simulink model "ES101A_DiagcMgrProxyX"  (R2013b)
settings: Solver=ode45  StartTime=0.0  StopTime=10.0  RelTol=1e-3
values from neighbouring files (symbols this model uses):
  DFTAGICNTR_CNT_U08 = DataDict.Constant    [ES101A_DiagcMgr_DataDict.m]
  DIAGCMGR_NTCINFOSTSTESTFAILD_CNT_U08 = DataDict.Constant    [ES101A_DiagcMgr_DataDict.m]
  DIAGCMGR_NTCINFOSTSTESTFAILDTHISIGNCYC_CNT_U08 = DataDict.Constant    [ES101A_DiagcMgr_DataDict.m]
  DIAGCMGR_NTCINFOSTSTESTNOTCMPLTHISIGNCYC_CNT_U08 = DataDict.Constant    [ES101A_DiagcMgr_DataDict.m]
  DiagcMgrFltResp = DataDict.Calibration    [ES101A_DiagcMgr_DataDict.m]
  DIAGCSTSDFTHWAG_CNT_U16 = DataDict.Constant    [ES101A_DiagcMgr_DataDict.m]
  DIAGCSTSDFTHWAGSERLCOMEXPRTVAL_CNT_U16 = DataDict.Constant    [ES101A_DiagcMgr_DataDict.m]
  DIAGCSTSDFTVEHSPD_CNT_U16 = DataDict.Constant    [ES101A_DiagcMgr_DataDict.m]
  DIAGCSTSININVAL_CNT_U16 = DataDict.Constant    [ES101A_DiagcMgr_DataDict.m]
  DIAGCSTSIVTR1INACTV_CNT_U16 = DataDict.Constant    [ES101A_DiagcMgr_DataDict.m]
  DIAGCSTSIVTR2INACTV_CNT_U16 = DataDict.Constant    [ES101A_DiagcMgr_DataDict.m]
  DIAGCSTSLIMDTPRFMNC_CNT_U16 = DataDict.Constant    [ES101A_DiagcMgr_DataDict.m]
  DIAGCSTSWHLIMBREJCTNDI_CNT_U16 = DataDict.Constant    [ES101A_DiagcMgr_DataDict.m]
  ELECGLBPRM_IVTRCNT_CNT_U08 = DataDict.ConfigParam    [ES101A_DiagcMgr_DataDict.m]
  MAXRAMPRATE_ULSPERSEC_F32 = DataDict.Constant    [ES101A_DiagcMgr_DataDict.m]
  MINRAMPRATE_ULSPERSEC_F32 = DataDict.Constant    [ES101A_DiagcMgr_DataDict.m]
  SCAMOTTQCMDTOONE_ULS_F32 = DataDict.Constant    [ES101A_DiagcMgr_DataDict.m]
  SCAMOTTQCMDTOZERO_ULS_F32 = DataDict.Constant    [ES101A_DiagcMgr_DataDict.m]
undefined symbols (not defined in the file or in its folder): ActvMotTqCmdSca, ActvRampRate, AgiCntr, DIAGCMGR_APPLIDXX_CNT_U08, DiagcMgrNtcMap, DiagcSts, NtcStInfo, Sts
libraries: simulink x21
(part 3 of 3)

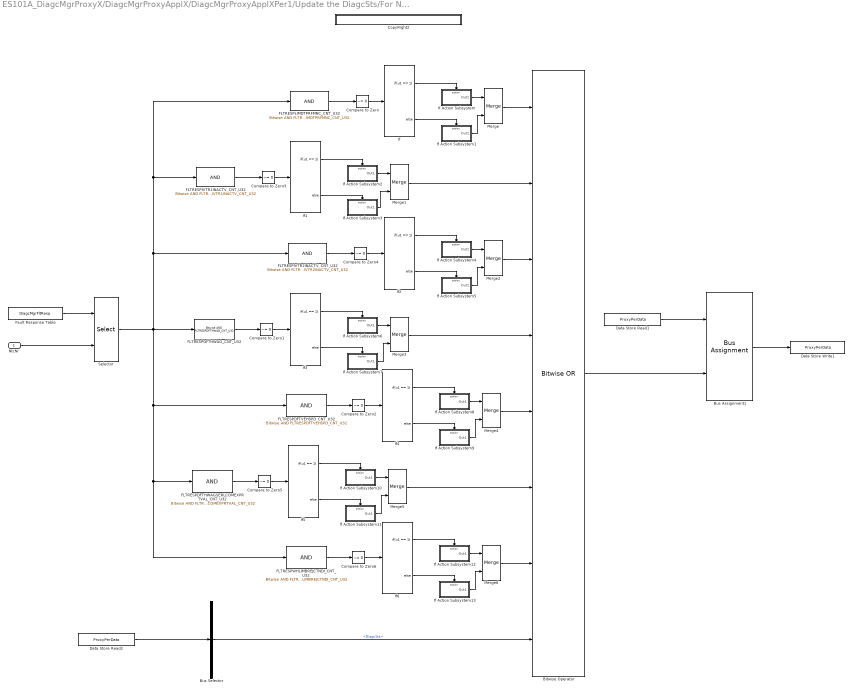
== system ES101A_DiagcMgrProxyX/DiagcMgrProxyApplX/DiagcMgrProxyApplXPer1/Update the DiagcSts/For Number of NTCs/Update DiagcSts and Ramp Response/Update Latest Values/ProcessDiagcSts ==
  NtcNr : Inport
  Bitwise Operator : simulink/Logic and Bit Operations/Bitwise Operator  logicop=OR  UseBitMask=off  NumInputPorts=8  BitMask=bin2dec('11011001')  BitMaskRealWorld=Stored Integer
  Bus Assignment1 : BusAssignment  AssignedSignals=DiagcSts
  Bus Selector : BusSelector  OutputSignals=DiagcSts
  Compare to Zero{,1..6} (7 alike) : simulink/Logic and Bit Operations/Compare To Zero  relop=~=  OutDataTypeStr=boolean
  CopyRight2 : Subsystem  Description=|  mask(Copyright Information){none=on}
      | Copyright info block.                                               
      |                                                                     
      | Place copyright information at the top of every subsystem in design.
      mask prompts: none "No parameters"
      mask help: Place copyright information at the top of every subsystem in design.
      mask Display:
      | NxtrConf = 'Nexteer Confidential';
      | 
      | sys = bdroot; %handle for the current model ("system")
      | first = get_param(sys,'Created');
      | first = first(end-3:end);  %year is last four digits
      | 
      | last = get_param(sys,'LastModifiedDate');
      | if isempty(last)
      |     last = datestr(now,'yyyy');
      | else
      |     last = last(end-3:end);
      | end
      | 
      | if strcmp(first,last)
      |     fprintf('%s -- Copyright %s Nexteer',NxtrConf,first)
      | else
      |     fprintf('%s -- %s%s- %s Nexteer',NxtrConf,char(169),first,last)
      | end
  Data Store Read1 : DataStoreRead  DataStoreName=ProxyPerData
  Data Store Read2 : DataStoreRead  DataStoreName=ProxyPerData
  Data Store Write1 : DataStoreWrite  DataStoreName=ProxyPerData
  FLTRESPDFTHWAGSERLCOMEXPRTVAL_CNT_U32 : simulink/Logic and Bit Operations/Bitwise Operator  logicop=AND  UseBitMask=on  BitMask=FLTRESPDFTHWAGSERLCOMEXPRTVAL_CNT_U32  BitMaskRealWorld=Stored Integer
  FLTRESPDFTHWAG_CNT_U32 : simulink/Logic and Bit Operations/Bitwise Operator  logicop=AND  UseBitMask=on  BitMask=FLTRESPDFTHWAG_CNT_U32  BitMaskRealWorld=Stored Integer
  FLTRESPDFTVEHSPD_CNT_U32 : simulink/Logic and Bit Operations/Bitwise Operator  logicop=AND  UseBitMask=on  BitMask=FLTRESPDFTVEHSPD_CNT_U32  BitMaskRealWorld=Stored Integer
  FLTRESPIVTR1INACTV_CNT_U32 : simulink/Logic and Bit Operations/Bitwise Operator  RequirementInfo={} %GIDa_f3ee0b00_0af4_4caf_9c85_8da4f7631b2d  logicop=AND  UseBitMask=on  BitMask=FLTRESPIVTR1INACTV_CNT_U32  BitMaskRealWorld=Stored Integer
  FLTRESPIVTR2INACTV_CNT_U32 : simulink/Logic and Bit Operations/Bitwise Operator  RequirementInfo={} %GIDa_c098454a_7649_4588_93b4_e3f297a380c8  logicop=AND  UseBitMask=on  BitMask=FLTRESPIVTR2INACTV_CNT_U32  BitMaskRealWorld=Stored Integer
  FLTRESPLIMDTPRFMNC_CNT_U32 : simulink/Logic and Bit Operations/Bitwise Operator  RequirementInfo={} %GIDa_abf10c00_ccc5_4fac_90af_e726bdec96c5  logicop=AND  UseBitMask=on  BitMask=FLTRESPLIMDTPRFMNC_CNT_U32  BitMaskRealWorld=Stored Integer
  FLTRESPWHLIMBREJCTNDI_CNT_U32 : simulink/Logic and Bit Operations/Bitwise Operator  logicop=AND  UseBitMask=on  BitMask=FLTRESPWHLIMBREJCTNDI_CNT_U32  BitMaskRealWorld=Stored Integer
  Fault Response Table : Constant  Value=DiagcMgrFltResp
  If{,1..6} (7 alike) : If  IfExpression=u1 == 1
  If Action Subsystem : Subsystem  TreatAsAtomicUnit=on
  If Action Subsystem1 : Subsystem  TreatAsAtomicUnit=on
  If Action Subsystem10 : Subsystem  TreatAsAtomicUnit=on
  If Action Subsystem11 : Subsystem  TreatAsAtomicUnit=on
  If Action Subsystem12 : Subsystem  TreatAsAtomicUnit=on
  If Action Subsystem13 : Subsystem  TreatAsAtomicUnit=on
  If Action Subsystem2 : Subsystem  TreatAsAtomicUnit=on
  If Action Subsystem3 : Subsystem  TreatAsAtomicUnit=on
  If Action Subsystem4 : Subsystem  TreatAsAtomicUnit=on
  If Action Subsystem5 : Subsystem  TreatAsAtomicUnit=on
  If Action Subsystem6 : Subsystem  TreatAsAtomicUnit=on
  If Action Subsystem7 : Subsystem  TreatAsAtomicUnit=on
  If Action Subsystem8 : Subsystem  TreatAsAtomicUnit=on
  If Action Subsystem9 : Subsystem  TreatAsAtomicUnit=on
  Merge{,1..6} (7 alike) : Merge
  Selector : Selector  IndexMode=Zero-based  InputPortWidth=512  IndexOptions=Index vector (port)  Indices=[1 3]  OutputSizes=1
  wires:
  Bitwise Operator/1 -> Bus Assignment1/2
  Bus Selector/1 -> Bitwise Operator/8  "<DiagcSts>"
  FLTRESPWHLIMBREJCTNDI_CNT_U32/1 -> Compare to Zero6/1
  If6/1 -> If Action Subsystem12/Action
  If6/2 -> If Action Subsystem13/Action
  If Action Subsystem12/1(Out1) -> Merge6/1
  If Action Subsystem13/1(Out1) -> Merge6/2
  Merge6/1 -> Bitwise Operator/7
  Compare to Zero6/1 -> If6/1
  FLTRESPDFTHWAGSERLCOMEXPRTVAL_CNT_U32/1 -> Compare to Zero5/1
  If5/1 -> If Action Subsystem10/Action
  If5/2 -> If Action Subsystem11/Action
  If Action Subsystem10/1(Out1) -> Merge5/1
  If Action Subsystem11/1(Out1) -> Merge5/2
  Merge5/1 -> Bitwise Operator/6
  Compare to Zero5/1 -> If5/1
  FLTRESPDFTVEHSPD_CNT_U32/1 -> Compare to Zero2/1
  If4/1 -> If Action Subsystem8/Action
  If4/2 -> If Action Subsystem9/Action
  If Action Subsystem8/1(Out1) -> Merge4/1
  If Action Subsystem9/1(Out1) -> Merge4/2
  Merge4/1 -> Bitwise Operator/5
  Compare to Zero2/1 -> If4/1
  FLTRESPDFTHWAG_CNT_U32/1 -> Compare to Zero1/1
  If3/1 -> If Action Subsystem6/Action
  If3/2 -> If Action Subsystem7/Action
  If Action Subsystem6/1(Out1) -> Merge3/1
  If Action Subsystem7/1(Out1) -> Merge3/2
  Merge3/1 -> Bitwise Operator/4
  Compare to Zero1/1 -> If3/1
  FLTRESPLIMDTPRFMNC_CNT_U32/1 -> Compare to Zero/1
  NtcNr/1 -> Selector/2
  Fault Response Table/1 -> Selector/1
  Selector/1 -> FLTRESPIVTR2INACTV_CNT_U32/1, FLTRESPIVTR1INACTV_CNT_U32/1, FLTRESPLIMDTPRFMNC_CNT_U32/1, FLTRESPDFTHWAG_CNT_U32/1, FLTRESPDFTVEHSPD_CNT_U32/1, FLTRESPDFTHWAGSERLCOMEXPRTVAL_CNT_U32/1, FLTRESPWHLIMBREJCTNDI_CNT_U32/1
  FLTRESPIVTR1INACTV_CNT_U32/1 -> Compare to Zero3/1
  FLTRESPIVTR2INACTV_CNT_U32/1 -> Compare to Zero4/1
  If/1 -> If Action Subsystem/Action
  If/2 -> If Action Subsystem1/Action
  Compare to Zero/1 -> If/1
  If Action Subsystem/1(Out1) -> Merge/1
  If Action Subsystem1/1(Out1) -> Merge/2
  Merge/1 -> Bitwise Operator/1
  If1/1 -> If Action Subsystem2/Action
  If1/2 -> If Action Subsystem3/Action
  If Action Subsystem2/1(Out1) -> Merge1/1
  If Action Subsystem3/1(Out1) -> Merge1/2
  Compare to Zero3/1 -> If1/1
  Merge1/1 -> Bitwise Operator/2
  If2/1 -> If Action Subsystem4/Action
  If2/2 -> If Action Subsystem5/Action
  If Action Subsystem4/1(Out1) -> Merge2/1
  If Action Subsystem5/1(Out1) -> Merge2/2
  Merge2/1 -> Bitwise Operator/3
  Compare to Zero4/1 -> If2/1
  Data Store Read1/1 -> Bus Assignment1/1
  Bus Assignment1/1 -> Data Store Write1/1
  Data Store Read2/1 -> Bus Selector/1

== system ES101A_DiagcMgrProxyX/DiagcMgrProxyApplX/DiagcMgrProxyApplXPer1/Update the DiagcSts/For Number of NTCs/Update DiagcSts and Ramp Response/Update Latest Values/ProcessRampResponse ==
  NtcNr : Inport
  Arithmetic Right Shift : ArithShift  BitShiftNumber=8  BitShiftDirection=Right
  ControlledShutdown Fault : Subsystem  RequirementInfo={} %GIDa_725417ca_b856_44d5_8006_295b90ff6843  TreatAsAtomicUnit=on
  CopyRight2 : Subsystem  Description=|  mask(Copyright Information){none=on}
      | Copyright info block.                                               
      |                                                                     
      | Place copyright information at the top of every subsystem in design.
      mask prompts: none "No parameters"
      mask help: Place copyright information at the top of every subsystem in design.
      mask Display:
      | NxtrConf = 'Nexteer Confidential';
      | 
      | sys = bdroot; %handle for the current model ("system")
      | first = get_param(sys,'Created');
      | first = first(end-3:end);  %year is last four digits
      | 
      | last = get_param(sys,'LastModifiedDate');
      | if isempty(last)
      |     last = datestr(now,'yyyy');
      | else
      |     last = last(end-3:end);
      | end
      | 
      | if strcmp(first,last)
      |     fprintf('%s -- Copyright %s Nexteer',NxtrConf,first)
      | else
      |     fprintf('%s -- %s%s- %s Nexteer',NxtrConf,char(169),first,last)
      | end
  FLTRESPRAMPBITS_CNT_U32 : simulink/Logic and Bit Operations/Bitwise Operator  logicop=AND  UseBitMask=on  BitMask=FLTRESPRAMPBITS_CNT_U32  BitMaskRealWorld=Stored Integer
  Fault Response Table : Constant  Value=DiagcMgrFltResp
  InformationOnly Fault : Subsystem  RequirementInfo={} %GIDa_ae2e5ce0_c467_4af9_b6e8_59d2bb6bb901  TreatAsAtomicUnit=on
  RapidShutdown Fault : Subsystem  RequirementInfo={} %GIDa_75af6023_41ae_4178_91eb_a83436bbf5a3  TreatAsAtomicUnit=on
  Selector1 : Selector  IndexMode=Zero-based  InputPortWidth=512  IndexOptions=Index vector (port)  Indices=[1 3]  OutputSizes=1
  Switch Case : SwitchCase  CaseConditions={15,14,13}
  TimedShutdown Fault : Subsystem  RequirementInfo={} %GIDa_32e9e7ae_b862_4160_9cdf_f89576b3a813  TreatAsAtomicUnit=on
  wires:
  Switch Case/4 -> TimedShutdown Fault/Action
  Switch Case/3 -> RapidShutdown Fault/Action
  Switch Case/2 -> ControlledShutdown Fault/Action
  Switch Case/1 -> InformationOnly Fault/Action
  Fault Response Table/1 -> Selector1/1
  Selector1/1 -> FLTRESPRAMPBITS_CNT_U32/1
  FLTRESPRAMPBITS_CNT_U32/1 -> Arithmetic Right Shift/1
  Arithmetic Right Shift/1 -> Switch Case/1, TimedShutdown Fault/1(FaultResponseRampBits)
  NtcNr/1 -> Selector1/2

== system ES101A_DiagcMgrProxyX/DiagcMgrProxyApplX/DiagcMgrProxyApplXPer1/Update the DiagcSts/For Number of NTCs/Update DiagcSts and Ramp Response/Update Latest Values/ProcessDiagcSts/CopyRight2 ==

== system ES101A_DiagcMgrProxyX/DiagcMgrProxyApplX/DiagcMgrProxyApplXPer1/Update the DiagcSts/For Number of NTCs/Update DiagcSts and Ramp Response/Update Latest Values/ProcessDiagcSts/If Action Subsystem ==
  Action Port : ActionPort
  Constant1 : Constant  Value=DIAGCSTSLIMDTPRFMNC_CNT_U16
  Out1 : Outport
  wires:
  Constant1/1 -> Out1/1

== system ES101A_DiagcMgrProxyX/DiagcMgrProxyApplX/DiagcMgrProxyApplXPer1/Update the DiagcSts/For Number of NTCs/Update DiagcSts and Ramp Response/Update Latest Values/ProcessDiagcSts/If Action Subsystem1 ==
  Action Port : ActionPort
  Constant1 : Constant  Value=0  OutDataTypeStr=uint16
  Out1 : Outport
  wires:
  Constant1/1 -> Out1/1

== system ES101A_DiagcMgrProxyX/DiagcMgrProxyApplX/DiagcMgrProxyApplXPer1/Update the DiagcSts/For Number of NTCs/Update DiagcSts and Ramp Response/Update Latest Values/ProcessDiagcSts/If Action Subsystem10 ==
  Action Port : ActionPort
  Constant1 : Constant  Value=DIAGCSTSDFTHWAGSERLCOMEXPRTVAL_CNT_U16
  Out1 : Outport
  wires:
  Constant1/1 -> Out1/1

== system ES101A_DiagcMgrProxyX/DiagcMgrProxyApplX/DiagcMgrProxyApplXPer1/Update the DiagcSts/For Number of NTCs/Update DiagcSts and Ramp Response/Update Latest Values/ProcessDiagcSts/If Action Subsystem11 ==
  Action Port : ActionPort
  Constant1 : Constant  Value=0  OutDataTypeStr=uint16
  Out1 : Outport
  wires:
  Constant1/1 -> Out1/1

== system ES101A_DiagcMgrProxyX/DiagcMgrProxyApplX/DiagcMgrProxyApplXPer1/Update the DiagcSts/For Number of NTCs/Update DiagcSts and Ramp Response/Update Latest Values/ProcessDiagcSts/If Action Subsystem12 ==
  Action Port : ActionPort
  Constant1 : Constant  Value=DIAGCSTSWHLIMBREJCTNDI_CNT_U16
  Out1 : Outport
  wires:
  Constant1/1 -> Out1/1

== system ES101A_DiagcMgrProxyX/DiagcMgrProxyApplX/DiagcMgrProxyApplXPer1/Update the DiagcSts/For Number of NTCs/Update DiagcSts and Ramp Response/Update Latest Values/ProcessDiagcSts/If Action Subsystem13 ==
  Action Port : ActionPort
  Constant1 : Constant  Value=0  OutDataTypeStr=uint16
  Out1 : Outport
  wires:
  Constant1/1 -> Out1/1

== system ES101A_DiagcMgrProxyX/DiagcMgrProxyApplX/DiagcMgrProxyApplXPer1/Update the DiagcSts/For Number of NTCs/Update DiagcSts and Ramp Response/Update Latest Values/ProcessDiagcSts/If Action Subsystem2 ==
  Action Port : ActionPort
  Constant1 : Constant  Value=DIAGCSTSIVTR1INACTV_CNT_U16
  Out1 : Outport
  wires:
  Constant1/1 -> Out1/1

== system ES101A_DiagcMgrProxyX/DiagcMgrProxyApplX/DiagcMgrProxyApplXPer1/Update the DiagcSts/For Number of NTCs/Update DiagcSts and Ramp Response/Update Latest Values/ProcessDiagcSts/If Action Subsystem3 ==
  Action Port : ActionPort
  Constant1 : Constant  Value=0  OutDataTypeStr=uint16
  Out1 : Outport
  wires:
  Constant1/1 -> Out1/1

== system ES101A_DiagcMgrProxyX/DiagcMgrProxyApplX/DiagcMgrProxyApplXPer1/Update the DiagcSts/For Number of NTCs/Update DiagcSts and Ramp Response/Update Latest Values/ProcessDiagcSts/If Action Subsystem4 ==
  Action Port : ActionPort
  Constant1 : Constant  Value=DIAGCSTSIVTR2INACTV_CNT_U16
  Out1 : Outport
  wires:
  Constant1/1 -> Out1/1

== system ES101A_DiagcMgrProxyX/DiagcMgrProxyApplX/DiagcMgrProxyApplXPer1/Update the DiagcSts/For Number of NTCs/Update DiagcSts and Ramp Response/Update Latest Values/ProcessDiagcSts/If Action Subsystem5 ==
  Action Port : ActionPort
  Constant1 : Constant  Value=0  OutDataTypeStr=uint16
  Out1 : Outport
  wires:
  Constant1/1 -> Out1/1

== system ES101A_DiagcMgrProxyX/DiagcMgrProxyApplX/DiagcMgrProxyApplXPer1/Update the DiagcSts/For Number of NTCs/Update DiagcSts and Ramp Response/Update Latest Values/ProcessDiagcSts/If Action Subsystem6 ==
  Action Port : ActionPort
  Constant1 : Constant  Value=DIAGCSTSDFTHWAG_CNT_U16
  Out1 : Outport
  wires:
  Constant1/1 -> Out1/1

== system ES101A_DiagcMgrProxyX/DiagcMgrProxyApplX/DiagcMgrProxyApplXPer1/Update the DiagcSts/For Number of NTCs/Update DiagcSts and Ramp Response/Update Latest Values/ProcessDiagcSts/If Action Subsystem7 ==
  Action Port : ActionPort
  Constant1 : Constant  Value=0  OutDataTypeStr=uint16
  Out1 : Outport
  wires:
  Constant1/1 -> Out1/1

== system ES101A_DiagcMgrProxyX/DiagcMgrProxyApplX/DiagcMgrProxyApplXPer1/Update the DiagcSts/For Number of NTCs/Update DiagcSts and Ramp Response/Update Latest Values/ProcessDiagcSts/If Action Subsystem8 ==
  Action Port : ActionPort
  Constant1 : Constant  Value=DIAGCSTSDFTVEHSPD_CNT_U16
  Out1 : Outport
  wires:
  Constant1/1 -> Out1/1

== system ES101A_DiagcMgrProxyX/DiagcMgrProxyApplX/DiagcMgrProxyApplXPer1/Update the DiagcSts/For Number of NTCs/Update DiagcSts and Ramp Response/Update Latest Values/ProcessDiagcSts/If Action Subsystem9 ==
  Action Port : ActionPort
  Constant1 : Constant  Value=0  OutDataTypeStr=uint16
  Out1 : Outport
  wires:
  Constant1/1 -> Out1/1

== system ES101A_DiagcMgrProxyX/DiagcMgrProxyApplX/DiagcMgrProxyApplXPer1/Update the DiagcSts/For Number of NTCs/Update DiagcSts and Ramp Response/Update Latest Values/ProcessRampResponse/ControlledShutdown Fault ==
  Action Port : ActionPort
  Bus Selector : BusSelector  OutputSignals=ActvMotTqCmdSca
  CopyRight2 : Subsystem  Description=|  mask(Copyright Information){none=on}
      | Copyright info block.                                               
      |                                                                     
      | Place copyright information at the top of every subsystem in design.
      mask prompts: none "No parameters"
      mask help: Place copyright information at the top of every subsystem in design.
      mask Display:
      | NxtrConf = 'Nexteer Confidential';
      | 
      | sys = bdroot; %handle for the current model ("system")
      | first = get_param(sys,'Created');
      | first = first(end-3:end);  %year is last four digits
      | 
      | last = get_param(sys,'LastModifiedDate');
      | if isempty(last)
      |     last = datestr(now,'yyyy');
      | else
      |     last = last(end-3:end);
      | end
      | 
      | if strcmp(first,last)
      |     fprintf('%s -- Copyright %s Nexteer',NxtrConf,first)
      | else
      |     fprintf('%s -- %s%s- %s Nexteer',NxtrConf,char(169),first,last)
      | end
  Data Store Read : DataStoreRead  DataStoreName=ProxyPerData
  Do Nothing : Subsystem  TreatAsAtomicUnit=on
  If : If  NumInputs=2  IfExpression=u1 < u2
  Scale Motor Torque Command to Zero1 : Constant  Value=SCAMOTTQCMDTOZERO_ULS_F32  OutDataTypeStr=single
  Update Scale : Subsystem  TreatAsAtomicUnit=on
  wires:
  Scale Motor Torque Command to Zero1/1 -> If/1
  Bus Selector/1 -> If/2  "<ActvMotTqCmdSca>"
  If/2 -> Do Nothing/Action
  If/1 -> Update Scale/Action
  Data Store Read/1 -> Bus Selector/1

== system ES101A_DiagcMgrProxyX/DiagcMgrProxyApplX/DiagcMgrProxyApplXPer1/Update the DiagcSts/For Number of NTCs/Update DiagcSts and Ramp Response/Update Latest Values/ProcessRampResponse/CopyRight2 ==

== system ES101A_DiagcMgrProxyX/DiagcMgrProxyApplX/DiagcMgrProxyApplXPer1/Update the DiagcSts/For Number of NTCs/Update DiagcSts and Ramp Response/Update Latest Values/ProcessRampResponse/InformationOnly Fault ==
  Action Port : ActionPort
  CopyRight2 : Subsystem  Description=|  mask(Copyright Information){none=on}
      | Copyright info block.                                               
      |                                                                     
      | Place copyright information at the top of every subsystem in design.
      mask prompts: none "No parameters"
      mask help: Place copyright information at the top of every subsystem in design.
      mask Display:
      | NxtrConf = 'Nexteer Confidential';
      | 
      | sys = bdroot; %handle for the current model ("system")
      | first = get_param(sys,'Created');
      | first = first(end-3:end);  %year is last four digits
      | 
      | last = get_param(sys,'LastModifiedDate');
      | if isempty(last)
      |     last = datestr(now,'yyyy');
      | else
      |     last = last(end-3:end);
      | end
      | 
      | if strcmp(first,last)
      |     fprintf('%s -- Copyright %s Nexteer',NxtrConf,first)
      | else
      |     fprintf('%s -- %s%s- %s Nexteer',NxtrConf,char(169),first,last)
      | end

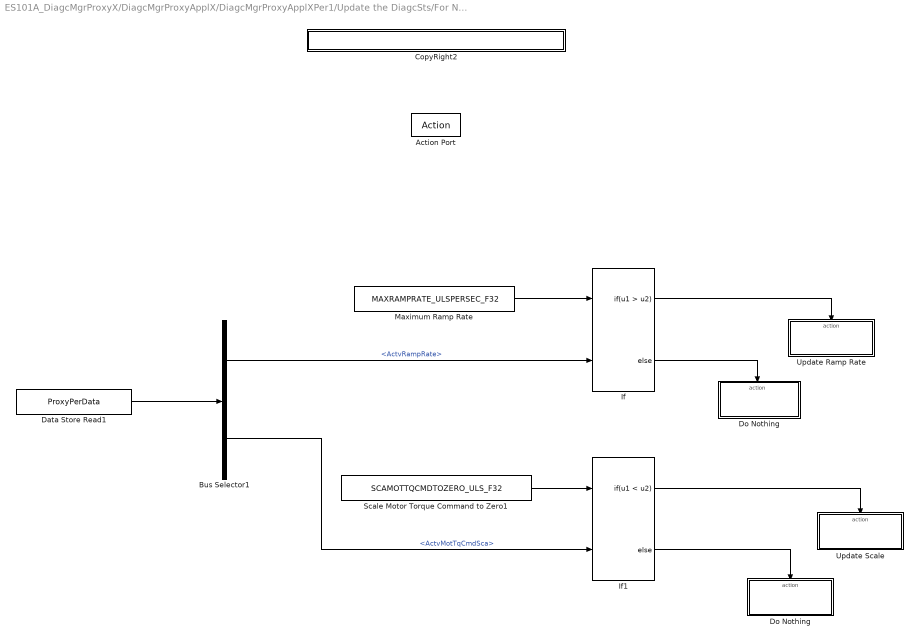
== system ES101A_DiagcMgrProxyX/DiagcMgrProxyApplX/DiagcMgrProxyApplXPer1/Update the DiagcSts/For Number of NTCs/Update DiagcSts and Ramp Response/Update Latest Values/ProcessRampResponse/RapidShutdown Fault ==
  Action Port : ActionPort
  Bus Selector1 : BusSelector  OutputSignals=ActvRampRate,ActvMotTqCmdSca
  CopyRight2 : Subsystem  Description=|  mask(Copyright Information){none=on}
      | Copyright info block.                                               
      |                                                                     
      | Place copyright information at the top of every subsystem in design.
      mask prompts: none "No parameters"
      mask help: Place copyright information at the top of every subsystem in design.
      mask Display:
      | NxtrConf = 'Nexteer Confidential';
      | 
      | sys = bdroot; %handle for the current model ("system")
      | first = get_param(sys,'Created');
      | first = first(end-3:end);  %year is last four digits
      | 
      | last = get_param(sys,'LastModifiedDate');
      | if isempty(last)
      |     last = datestr(now,'yyyy');
      | else
      |     last = last(end-3:end);
      | end
      | 
      | if strcmp(first,last)
      |     fprintf('%s -- Copyright %s Nexteer',NxtrConf,first)
      | else
      |     fprintf('%s -- %s%s- %s Nexteer',NxtrConf,char(169),first,last)
      | end
  Data Store Read1 : DataStoreRead  DataStoreName=ProxyPerData
  Do Nothing : Subsystem  TreatAsAtomicUnit=on
  "Do Nothing " : Subsystem  TreatAsAtomicUnit=on
  If : If  NumInputs=2  IfExpression=u1 > u2
  If1 : If  NumInputs=2  IfExpression=u1 < u2
  Maximum Ramp Rate : Constant  Value=MAXRAMPRATE_ULSPERSEC_F32  OutDataTypeStr=single
  Scale Motor Torque Command to Zero1 : Constant  Value=SCAMOTTQCMDTOZERO_ULS_F32  OutDataTypeStr=single
  Update Ramp Rate : Subsystem  TreatAsAtomicUnit=on
  Update Scale : Subsystem  TreatAsAtomicUnit=on
  wires:
  Maximum Ramp Rate/1 -> If/1
  Bus Selector1/1 -> If/2  "<ActvRampRate>"
  If/2 -> "Do Nothing "/Action
  If/1 -> Update Ramp Rate/Action
  Scale Motor Torque Command to Zero1/1 -> If1/1
  If1/2 -> Do Nothing/Action
  If1/1 -> Update Scale/Action
  Data Store Read1/1 -> Bus Selector1/1
  Bus Selector1/2 -> If1/2  "<ActvMotTqCmdSca>"

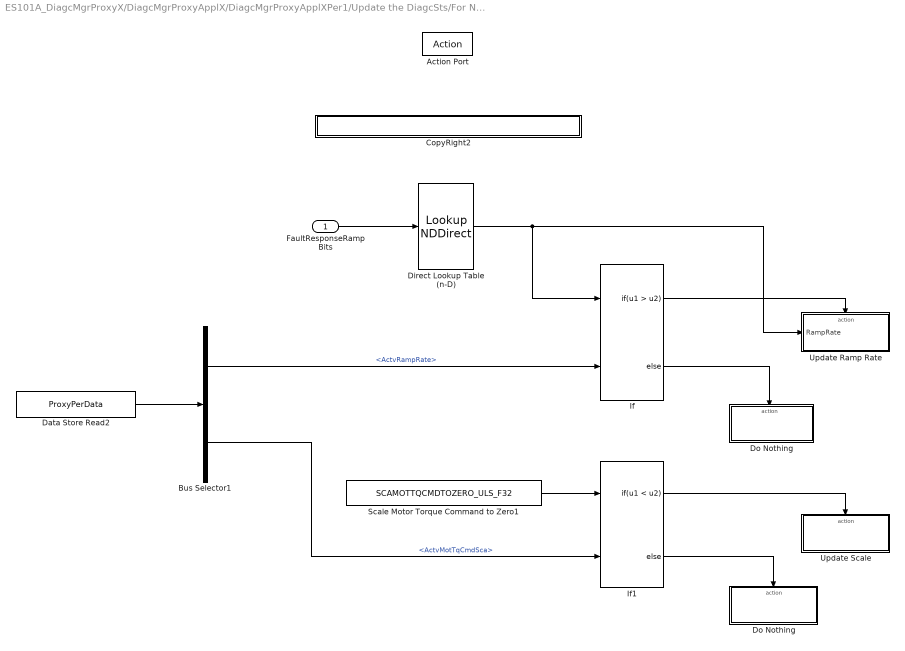
== system ES101A_DiagcMgrProxyX/DiagcMgrProxyApplX/DiagcMgrProxyApplXPer1/Update the DiagcSts/For Number of NTCs/Update DiagcSts and Ramp Response/Update Latest Values/ProcessRampResponse/TimedShutdown Fault ==
  FaultResponseRampBits : Inport
  Action Port : ActionPort
  Bus Selector1 : BusSelector  OutputSignals=ActvRampRate,ActvMotTqCmdSca
  CopyRight2 : Subsystem  Description=|  mask(Copyright Information){none=on}
      | Copyright info block.                                               
      |                                                                     
      | Place copyright information at the top of every subsystem in design.
      mask prompts: none "No parameters"
      mask help: Place copyright information at the top of every subsystem in design.
      mask Display:
      | NxtrConf = 'Nexteer Confidential';
      | 
      | sys = bdroot; %handle for the current model ("system")
      | first = get_param(sys,'Created');
      | first = first(end-3:end);  %year is last four digits
      | 
      | last = get_param(sys,'LastModifiedDate');
      | if isempty(last)
      |     last = datestr(now,'yyyy');
      | else
      |     last = last(end-3:end);
      | end
      | 
      | if strcmp(first,last)
      |     fprintf('%s -- Copyright %s Nexteer',NxtrConf,first)
      | else
      |     fprintf('%s -- %s%s- %s Nexteer',NxtrConf,char(169),first,last)
      | end
  Data Store Read2 : DataStoreRead  DataStoreName=ProxyPerData
  Direct Lookup Table (n-D) : LookupNDDirect  NumberOfTableDimensions=1  Table=[0.1,0.125,0.1428,0.1667,0.2,0.25,0.333,0.5,1,2,3.333,10,500]  TableDataTypeStr=single
  Do Nothing : Subsystem  TreatAsAtomicUnit=on
  "Do Nothing " : Subsystem  TreatAsAtomicUnit=on
  If : If  NumInputs=2  IfExpression=u1 > u2
  If1 : If  NumInputs=2  IfExpression=u1 < u2
  Scale Motor Torque Command to Zero1 : Constant  Value=SCAMOTTQCMDTOZERO_ULS_F32  OutDataTypeStr=single
  Update Ramp Rate : Subsystem  TreatAsAtomicUnit=on
  Update Scale : Subsystem  TreatAsAtomicUnit=on
  wires:
  Direct Lookup Table (n-D)/1 -> If/1, Update Ramp Rate/1(RampRate)
  Scale Motor Torque Command to Zero1/1 -> If1/1
  If1/2 -> Do Nothing/Action
  If1/1 -> Update Scale/Action
  If/2 -> "Do Nothing "/Action
  If/1 -> Update Ramp Rate/Action
  FaultResponseRampBits/1 -> Direct Lookup Table (n-D)/1
  Bus Selector1/1 -> If/2  "<ActvRampRate>"
  Data Store Read2/1 -> Bus Selector1/1
  Bus Selector1/2 -> If1/2  "<ActvMotTqCmdSca>"

== system ES101A_DiagcMgrProxyX/DiagcMgrProxyApplX/DiagcMgrProxyApplXPer1/Update the DiagcSts/For Number of NTCs/Update DiagcSts and Ramp Response/Update Latest Values/ProcessRampResponse/ControlledShutdown Fault/CopyRight2 ==

== system ES101A_DiagcMgrProxyX/DiagcMgrProxyApplX/DiagcMgrProxyApplXPer1/Update the DiagcSts/For Number of NTCs/Update DiagcSts and Ramp Response/Update Latest Values/ProcessRampResponse/ControlledShutdown Fault/Do Nothing ==
  Action Port : ActionPort
  CopyRight2 : Subsystem  Description=|  mask(Copyright Information){none=on}
      | Copyright info block.                                               
      |                                                                     
      | Place copyright information at the top of every subsystem in design.
      mask prompts: none "No parameters"
      mask help: Place copyright information at the top of every subsystem in design.
      mask Display:
      | NxtrConf = 'Nexteer Confidential';
      | 
      | sys = bdroot; %handle for the current model ("system")
      | first = get_param(sys,'Created');
      | first = first(end-3:end);  %year is last four digits
      | 
      | last = get_param(sys,'LastModifiedDate');
      | if isempty(last)
      |     last = datestr(now,'yyyy');
      | else
      |     last = last(end-3:end);
      | end
      | 
      | if strcmp(first,last)
      |     fprintf('%s -- Copyright %s Nexteer',NxtrConf,first)
      | else
      |     fprintf('%s -- %s%s- %s Nexteer',NxtrConf,char(169),first,last)
      | end

== system ES101A_DiagcMgrProxyX/DiagcMgrProxyApplX/DiagcMgrProxyApplXPer1/Update the DiagcSts/For Number of NTCs/Update DiagcSts and Ramp Response/Update Latest Values/ProcessRampResponse/ControlledShutdown Fault/Update Scale ==
  Action Port : ActionPort
  Bus Assignment1 : BusAssignment  AssignedSignals=ActvMotTqCmdSca
  CopyRight2 : Subsystem  Description=|  mask(Copyright Information){none=on}
      | Copyright info block.                                               
      |                                                                     
      | Place copyright information at the top of every subsystem in design.
      mask prompts: none "No parameters"
      mask help: Place copyright information at the top of every subsystem in design.
      mask Display:
      | NxtrConf = 'Nexteer Confidential';
      | 
      | sys = bdroot; %handle for the current model ("system")
      | first = get_param(sys,'Created');
      | first = first(end-3:end);  %year is last four digits
      | 
      | last = get_param(sys,'LastModifiedDate');
      | if isempty(last)
      |     last = datestr(now,'yyyy');
      | else
      |     last = last(end-3:end);
      | end
      | 
      | if strcmp(first,last)
      |     fprintf('%s -- Copyright %s Nexteer',NxtrConf,first)
      | else
      |     fprintf('%s -- %s%s- %s Nexteer',NxtrConf,char(169),first,last)
      | end
  Data Store Read : DataStoreRead  DataStoreName=ProxyPerData
  Data Store Write : DataStoreWrite  DataStoreName=ProxyPerData
  Scale Motor Torque Command to Zero : Constant  Value=SCAMOTTQCMDTOZERO_ULS_F32  OutDataTypeStr=single
  wires:
  Data Store Read/1 -> Bus Assignment1/1
  Bus Assignment1/1 -> Data Store Write/1
  Scale Motor Torque Command to Zero/1 -> Bus Assignment1/2

== system ES101A_DiagcMgrProxyX/DiagcMgrProxyApplX/DiagcMgrProxyApplXPer1/Update the DiagcSts/For Number of NTCs/Update DiagcSts and Ramp Response/Update Latest Values/ProcessRampResponse/InformationOnly Fault/CopyRight2 ==

== system ES101A_DiagcMgrProxyX/DiagcMgrProxyApplX/DiagcMgrProxyApplXPer1/Update the DiagcSts/For Number of NTCs/Update DiagcSts and Ramp Response/Update Latest Values/ProcessRampResponse/RapidShutdown Fault/CopyRight2 ==

== system ES101A_DiagcMgrProxyX/DiagcMgrProxyApplX/DiagcMgrProxyApplXPer1/Update the DiagcSts/For Number of NTCs/Update DiagcSts and Ramp Response/Update Latest Values/ProcessRampResponse/RapidShutdown Fault/Do Nothing ==
  Action Port : ActionPort
  CopyRight2 : Subsystem  Description=|  mask(Copyright Information){none=on}
      | Copyright info block.                                               
      |                                                                     
      | Place copyright information at the top of every subsystem in design.
      mask prompts: none "No parameters"
      mask help: Place copyright information at the top of every subsystem in design.
      mask Display:
      | NxtrConf = 'Nexteer Confidential';
      | 
      | sys = bdroot; %handle for the current model ("system")
      | first = get_param(sys,'Created');
      | first = first(end-3:end);  %year is last four digits
      | 
      | last = get_param(sys,'LastModifiedDate');
      | if isempty(last)
      |     last = datestr(now,'yyyy');
      | else
      |     last = last(end-3:end);
      | end
      | 
      | if strcmp(first,last)
      |     fprintf('%s -- Copyright %s Nexteer',NxtrConf,first)
      | else
      |     fprintf('%s -- %s%s- %s Nexteer',NxtrConf,char(169),first,last)
      | end

== system ES101A_DiagcMgrProxyX/DiagcMgrProxyApplX/DiagcMgrProxyApplXPer1/Update the DiagcSts/For Number of NTCs/Update DiagcSts and Ramp Response/Update Latest Values/ProcessRampResponse/RapidShutdown Fault/Do Nothing  ==
  Action Port : ActionPort
  CopyRight2 : Subsystem  Description=|  mask(Copyright Information){none=on}
      | Copyright info block.                                               
      |                                                                     
      | Place copyright information at the top of every subsystem in design.
      mask prompts: none "No parameters"
      mask help: Place copyright information at the top of every subsystem in design.
      mask Display:
      | NxtrConf = 'Nexteer Confidential';
      | 
      | sys = bdroot; %handle for the current model ("system")
      | first = get_param(sys,'Created');
      | first = first(end-3:end);  %year is last four digits
      | 
      | last = get_param(sys,'LastModifiedDate');
      | if isempty(last)
      |     last = datestr(now,'yyyy');
      | else
      |     last = last(end-3:end);
      | end
      | 
      | if strcmp(first,last)
      |     fprintf('%s -- Copyright %s Nexteer',NxtrConf,first)
      | else
      |     fprintf('%s -- %s%s- %s Nexteer',NxtrConf,char(169),first,last)
      | end

== system ES101A_DiagcMgrProxyX/DiagcMgrProxyApplX/DiagcMgrProxyApplXPer1/Update the DiagcSts/For Number of NTCs/Update DiagcSts and Ramp Response/Update Latest Values/ProcessRampResponse/RapidShutdown Fault/Update Ramp Rate ==
  Action Port : ActionPort
  Bus Assignment1 : BusAssignment  AssignedSignals=ActvRampRate
  CopyRight2 : Subsystem  Description=|  mask(Copyright Information){none=on}
      | Copyright info block.                                               
      |                                                                     
      | Place copyright information at the top of every subsystem in design.
      mask prompts: none "No parameters"
      mask help: Place copyright information at the top of every subsystem in design.
      mask Display:
      | NxtrConf = 'Nexteer Confidential';
      | 
      | sys = bdroot; %handle for the current model ("system")
      | first = get_param(sys,'Created');
      | first = first(end-3:end);  %year is last four digits
      | 
      | last = get_param(sys,'LastModifiedDate');
      | if isempty(last)
      |     last = datestr(now,'yyyy');
      | else
      |     last = last(end-3:end);
      | end
      | 
      | if strcmp(first,last)
      |     fprintf('%s -- Copyright %s Nexteer',NxtrConf,first)
      | else
      |     fprintf('%s -- %s%s- %s Nexteer',NxtrConf,char(169),first,last)
      | end
  Data Store Read : DataStoreRead  DataStoreName=ProxyPerData
  Data Store Write : DataStoreWrite  DataStoreName=ProxyPerData
  Maximum Ramp Rate : Constant  Value=MAXRAMPRATE_ULSPERSEC_F32  OutDataTypeStr=single
  wires:
  Maximum Ramp Rate/1 -> Bus Assignment1/2
  Data Store Read/1 -> Bus Assignment1/1
  Bus Assignment1/1 -> Data Store Write/1

== system ES101A_DiagcMgrProxyX/DiagcMgrProxyApplX/DiagcMgrProxyApplXPer1/Update the DiagcSts/For Number of NTCs/Update DiagcSts and Ramp Response/Update Latest Values/ProcessRampResponse/RapidShutdown Fault/Update Scale ==
  Action Port : ActionPort
  Bus Assignment1 : BusAssignment  AssignedSignals=ActvMotTqCmdSca
  CopyRight2 : Subsystem  Description=|  mask(Copyright Information){none=on}
      | Copyright info block.                                               
      |                                                                     
      | Place copyright information at the top of every subsystem in design.
      mask prompts: none "No parameters"
      mask help: Place copyright information at the top of every subsystem in design.
      mask Display:
      | NxtrConf = 'Nexteer Confidential';
      | 
      | sys = bdroot; %handle for the current model ("system")
      | first = get_param(sys,'Created');
      | first = first(end-3:end);  %year is last four digits
      | 
      | last = get_param(sys,'LastModifiedDate');
      | if isempty(last)
      |     last = datestr(now,'yyyy');
      | else
      |     last = last(end-3:end);
      | end
      | 
      | if strcmp(first,last)
      |     fprintf('%s -- Copyright %s Nexteer',NxtrConf,first)
      | else
      |     fprintf('%s -- %s%s- %s Nexteer',NxtrConf,char(169),first,last)
      | end
  Data Store Read : DataStoreRead  DataStoreName=ProxyPerData
  Data Store Write : DataStoreWrite  DataStoreName=ProxyPerData
  Scale Motor Torque Command to Zero : Constant  Value=SCAMOTTQCMDTOZERO_ULS_F32  OutDataTypeStr=single
  wires:
  Data Store Read/1 -> Bus Assignment1/1
  Bus Assignment1/1 -> Data Store Write/1
  Scale Motor Torque Command to Zero/1 -> Bus Assignment1/2

== system ES101A_DiagcMgrProxyX/DiagcMgrProxyApplX/DiagcMgrProxyApplXPer1/Update the DiagcSts/For Number of NTCs/Update DiagcSts and Ramp Response/Update Latest Values/ProcessRampResponse/TimedShutdown Fault/CopyRight2 ==

== system ES101A_DiagcMgrProxyX/DiagcMgrProxyApplX/DiagcMgrProxyApplXPer1/Update the DiagcSts/For Number of NTCs/Update DiagcSts and Ramp Response/Update Latest Values/ProcessRampResponse/TimedShutdown Fault/Do Nothing ==
  Action Port : ActionPort
  CopyRight2 : Subsystem  Description=|  mask(Copyright Information){none=on}
      | Copyright info block.                                               
      |                                                                     
      | Place copyright information at the top of every subsystem in design.
      mask prompts: none "No parameters"
      mask help: Place copyright information at the top of every subsystem in design.
      mask Display:
      | NxtrConf = 'Nexteer Confidential';
      | 
      | sys = bdroot; %handle for the current model ("system")
      | first = get_param(sys,'Created');
      | first = first(end-3:end);  %year is last four digits
      | 
      | last = get_param(sys,'LastModifiedDate');
      | if isempty(last)
      |     last = datestr(now,'yyyy');
      | else
      |     last = last(end-3:end);
      | end
      | 
      | if strcmp(first,last)
      |     fprintf('%s -- Copyright %s Nexteer',NxtrConf,first)
      | else
      |     fprintf('%s -- %s%s- %s Nexteer',NxtrConf,char(169),first,last)
      | end

== system ES101A_DiagcMgrProxyX/DiagcMgrProxyApplX/DiagcMgrProxyApplXPer1/Update the DiagcSts/For Number of NTCs/Update DiagcSts and Ramp Response/Update Latest Values/ProcessRampResponse/TimedShutdown Fault/Do Nothing  ==
  Action Port : ActionPort
  CopyRight2 : Subsystem  Description=|  mask(Copyright Information){none=on}
      | Copyright info block.                                               
      |                                                                     
      | Place copyright information at the top of every subsystem in design.
      mask prompts: none "No parameters"
      mask help: Place copyright information at the top of every subsystem in design.
      mask Display:
      | NxtrConf = 'Nexteer Confidential';
      | 
      | sys = bdroot; %handle for the current model ("system")
      | first = get_param(sys,'Created');
      | first = first(end-3:end);  %year is last four digits
      | 
      | last = get_param(sys,'LastModifiedDate');
      | if isempty(last)
      |     last = datestr(now,'yyyy');
      | else
      |     last = last(end-3:end);
      | end
      | 
      | if strcmp(first,last)
      |     fprintf('%s -- Copyright %s Nexteer',NxtrConf,first)
      | else
      |     fprintf('%s -- %s%s- %s Nexteer',NxtrConf,char(169),first,last)
      | end

== system ES101A_DiagcMgrProxyX/DiagcMgrProxyApplX/DiagcMgrProxyApplXPer1/Update the DiagcSts/For Number of NTCs/Update DiagcSts and Ramp Response/Update Latest Values/ProcessRampResponse/TimedShutdown Fault/Update Ramp Rate ==
  RampRate : Inport
  Action Port : ActionPort
  Bus Assignment1 : BusAssignment  AssignedSignals=ActvRampRate
  CopyRight2 : Subsystem  Description=|  mask(Copyright Information){none=on}
      | Copyright info block.                                               
      |                                                                     
      | Place copyright information at the top of every subsystem in design.
      mask prompts: none "No parameters"
      mask help: Place copyright information at the top of every subsystem in design.
      mask Display:
      | NxtrConf = 'Nexteer Confidential';
      | 
      | sys = bdroot; %handle for the current model ("system")
      | first = get_param(sys,'Created');
      | first = first(end-3:end);  %year is last four digits
      | 
      | last = get_param(sys,'LastModifiedDate');
      | if isempty(last)
      |     last = datestr(now,'yyyy');
      | else
      |     last = last(end-3:end);
      | end
      | 
      | if strcmp(first,last)
      |     fprintf('%s -- Copyright %s Nexteer',NxtrConf,first)
      | else
      |     fprintf('%s -- %s%s- %s Nexteer',NxtrConf,char(169),first,last)
      | end
  Data Store Read : DataStoreRead  DataStoreName=ProxyPerData
  Data Store Write : DataStoreWrite  DataStoreName=ProxyPerData
  wires:
  RampRate/1 -> Bus Assignment1/2
  Data Store Read/1 -> Bus Assignment1/1
  Bus Assignment1/1 -> Data Store Write/1

== system ES101A_DiagcMgrProxyX/DiagcMgrProxyApplX/DiagcMgrProxyApplXPer1/Update the DiagcSts/For Number of NTCs/Update DiagcSts and Ramp Response/Update Latest Values/ProcessRampResponse/TimedShutdown Fault/Update Scale ==
  Action Port : ActionPort
  Bus Assignment1 : BusAssignment  AssignedSignals=ActvMotTqCmdSca
  CopyRight2 : Subsystem  Description=|  mask(Copyright Information){none=on}
      | Copyright info block.                                               
      |                                                                     
      | Place copyright information at the top of every subsystem in design.
      mask prompts: none "No parameters"
      mask help: Place copyright information at the top of every subsystem in design.
      mask Display:
      | NxtrConf = 'Nexteer Confidential';
      | 
      | sys = bdroot; %handle for the current model ("system")
      | first = get_param(sys,'Created');
      | first = first(end-3:end);  %year is last four digits
      | 
      | last = get_param(sys,'LastModifiedDate');
      | if isempty(last)
      |     last = datestr(now,'yyyy');
      | else
      |     last = last(end-3:end);
      | end
      | 
      | if strcmp(first,last)
      |     fprintf('%s -- Copyright %s Nexteer',NxtrConf,first)
      | else
      |     fprintf('%s -- %s%s- %s Nexteer',NxtrConf,char(169),first,last)
      | end
  Data Store Read : DataStoreRead  DataStoreName=ProxyPerData
  Data Store Write : DataStoreWrite  DataStoreName=ProxyPerData
  Scale Motor Torque Command to Zero : Constant  Value=SCAMOTTQCMDTOZERO_ULS_F32  OutDataTypeStr=single
  wires:
  Data Store Read/1 -> Bus Assignment1/1
  Bus Assignment1/1 -> Data Store Write/1
  Scale Motor Torque Command to Zero/1 -> Bus Assignment1/2

== system ES101A_DiagcMgrProxyX/DiagcMgrProxyApplX/DiagcMgrProxyApplXPer1/Update the DiagcSts/For Number of NTCs/Update DiagcSts and Ramp Response/Update Latest Values/ProcessRampResponse/ControlledShutdown Fault/Do Nothing/CopyRight2 ==

== system ES101A_DiagcMgrProxyX/DiagcMgrProxyApplX/DiagcMgrProxyApplXPer1/Update the DiagcSts/For Number of NTCs/Update DiagcSts and Ramp Response/Update Latest Values/ProcessRampResponse/ControlledShutdown Fault/Update Scale/CopyRight2 ==

== system ES101A_DiagcMgrProxyX/DiagcMgrProxyApplX/DiagcMgrProxyApplXPer1/Update the DiagcSts/For Number of NTCs/Update DiagcSts and Ramp Response/Update Latest Values/ProcessRampResponse/RapidShutdown Fault/Do Nothing/CopyRight2 ==

== system ES101A_DiagcMgrProxyX/DiagcMgrProxyApplX/DiagcMgrProxyApplXPer1/Update the DiagcSts/For Number of NTCs/Update DiagcSts and Ramp Response/Update Latest Values/ProcessRampResponse/RapidShutdown Fault/Do Nothing /CopyRight2 ==

== system ES101A_DiagcMgrProxyX/DiagcMgrProxyApplX/DiagcMgrProxyApplXPer1/Update the DiagcSts/For Number of NTCs/Update DiagcSts and Ramp Response/Update Latest Values/ProcessRampResponse/RapidShutdown Fault/Update Ramp Rate/CopyRight2 ==

== system ES101A_DiagcMgrProxyX/DiagcMgrProxyApplX/DiagcMgrProxyApplXPer1/Update the DiagcSts/For Number of NTCs/Update DiagcSts and Ramp Response/Update Latest Values/ProcessRampResponse/RapidShutdown Fault/Update Scale/CopyRight2 ==

== system ES101A_DiagcMgrProxyX/DiagcMgrProxyApplX/DiagcMgrProxyApplXPer1/Update the DiagcSts/For Number of NTCs/Update DiagcSts and Ramp Response/Update Latest Values/ProcessRampResponse/TimedShutdown Fault/Do Nothing/CopyRight2 ==

== system ES101A_DiagcMgrProxyX/DiagcMgrProxyApplX/DiagcMgrProxyApplXPer1/Update the DiagcSts/For Number of NTCs/Update DiagcSts and Ramp Response/Update Latest Values/ProcessRampResponse/TimedShutdown Fault/Do Nothing /CopyRight2 ==

== system ES101A_DiagcMgrProxyX/DiagcMgrProxyApplX/DiagcMgrProxyApplXPer1/Update the DiagcSts/For Number of NTCs/Update DiagcSts and Ramp Response/Update Latest Values/ProcessRampResponse/TimedShutdown Fault/Update Ramp Rate/CopyRight2 ==

== system ES101A_DiagcMgrProxyX/DiagcMgrProxyApplX/DiagcMgrProxyApplXPer1/Update the DiagcSts/For Number of NTCs/Update DiagcSts and Ramp Response/Update Latest Values/ProcessRampResponse/TimedShutdown Fault/Update Scale/CopyRight2 ==
